simulink model "fitz_relay"  (R2015a)
settings: Solver=ode45  StartTime=0.0  StopTime=tmax  RelTol=1e-3
values from neighbouring files (symbols this model uses):
  A = gamma-alpha    (= 2.5)    [added_current_fitz_relay.m]    (also in example_1.m = [0 1 1; 0 -1 6; 0 0 -1]; goodwin_prediction.m = [-1 0 0 ; 1 -1 0; 0 1 -1]; new_fitz_relay.m = -1.5; relay_fitz_nagumo.m)
  B = 1    [added_current_fitz_relay.m]    (also in example_1.m = [1; 6; 6]; goodwin_prediction.m = [1; 0 ; 0]; new_fitz_relay.m; relay_fitz_nagumo.m)
  C = 1    [added_current_fitz_relay.m]    (also in example_1.m = [1 0 0]; goodwin_prediction.m = [0 0 1]; new_fitz_relay.m; relay_fitz_nagumo.m)
  D = 0    [added_current_fitz_relay.m]    (also in goodwin_prediction.m; new_fitz_relay.m; relay_fitz_nagumo.m; test_goodwin.m)
  d2 = 0.25    [added_current_fitz_relay.m]    (also in epsilon_sensitivity_to_d1_d2.m = 0.2829; goodwin_prediction.m = 0; new_fitz_relay.m; relay_fitz_nagumo.m = abs(mean([a(2,2) a(2,4)])))
  epsilon_1 = out(1)    [added_current_fitz_relay.m]    (also in example_1.m = -1; new_fitz_relay.m = -(epsilon_1 - I_app); relay_fitz_nagumo.m = a(1,1))
  epsilon_2 = out(2)    [added_current_fitz_relay.m]    (also in example_1.m = 1; new_fitz_relay.m = -(epsilon_2 - I_app); relay_fitz_nagumo.m = a(1,3))
  X0 = a1    [added_current_fitz_relay.m]    (also in example_1.m; new_fitz_relay.m; relay_fitz_nagumo.m = a2; test_goodwin.m = -a1)
settings Model: Creator=RAK  LastModifiedBy=RAK

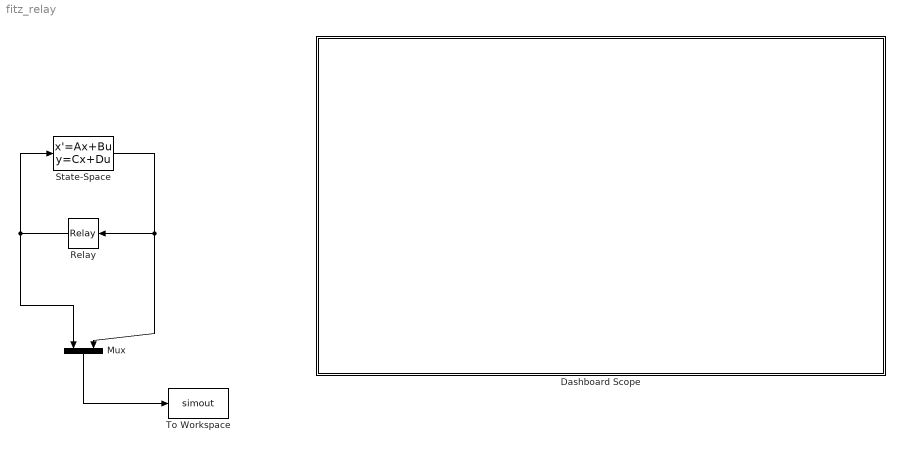
== system fitz_relay ==
  Dashboard Scope : Subsystem  DialogController=hmiCreateDDGDialog  IsWebBlock=on  mask(MathWorksWebBlock){webBlockId=a9f662bf-b164-4a37-8d9b-2b224a334fd7, webBlockType=sdiscope, ShowInitialText=on, HMISrcModelName=fitz_relay}
      mask prompts: webBlockId "WebBlock Id"; webBlockType "WebBlock Type"; HMISrcModelName "Source Model"
      mask Help: helpview([docroot '/mapfiles/simulink.map'], 'hmi_scope')
      mask Display:
      | if strcmp(get_param(bdroot(gcb),'BlockDiagramType'), 'library')
      |     image([(matlabroot) '/toolbox/simulink/hmi/icons/DashboardScope.png']);
      | end
  Mux : Mux  Inputs=2
  Relay : Relay  OnSwitchValue=epsilon_2  OffSwitchValue=epsilon_1  OnOutputValue=-d2  OffOutputValue=d1
  State-Space : StateSpace  A=A  B=B  C=C  D=D  X0=X0
  To Workspace : ToWorkspace  VariableName=simout  SaveFormat=Timeseries  SampleTime=-1
  wires:
  State-Space/1 -> Mux/2, Relay/1
  Relay/1 -> State-Space/1, Mux/1
  Mux/1 -> To Workspace/1

== system fitz_relay/Dashboard Scope ==
